simulink model "ejer1"  (R2015b)
settings: Solver=VariableStepAuto  StartTime=0.0  StopTime=10.0  RelTol=1e-3
libraries: powerlib x8
settings Model: Creator=xmax1946  LastModifiedBy=xmax1946

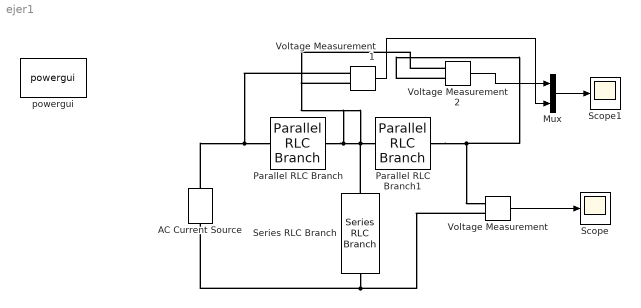
== system ejer1 ==
  AC Current Source : powerlib/Electrical Sources/AC Current Source  Amplitude=1  Phase=0  Frequency=.159  SampleTime=0  Measurements=None
  Mux : Mux  Inputs=2
  Parallel RLC Branch : powerlib/Elements/Parallel RLC Branch  LConnTagsString=a  RConnTagsString=__new0  BranchType=RC  Resistance=10  Inductance=1e-3  SetiL0=off  InitialCurrent=0  Capacitance=1  Setx0=on  InitialVoltage=100  Measurements=None
  Parallel RLC Branch1 : powerlib/Elements/Parallel RLC Branch  LConnTagsString=a  RConnTagsString=__new0  BranchType=RC  Resistance=1  Inductance=1e-3  SetiL0=off  InitialCurrent=0  Capacitance=2  Setx0=on  InitialVoltage=1  Measurements=None
  Scope : Scope
  Scope1 : Scope
  Series RLC Branch : powerlib/Elements/Series RLC Branch  LConnTagsString=__new0  RConnTagsString=__new0  BranchType=R  Resistance=1  Inductance=1e-3  SetiL0=off  InitialCurrent=0  Capacitance=1e-6  Setx0=off  InitialVoltage=0  Measurements=None
  Voltage Measurement : powerlib/Measurements/Voltage Measurement  PhasorSimulation=off  OutputType=Complex  PSBequivalent=0
  Voltage Measurement1 : powerlib/Measurements/Voltage Measurement  PhasorSimulation=off  OutputType=Complex  PSBequivalent=0
  Voltage Measurement2 : powerlib/Measurements/Voltage Measurement  PhasorSimulation=off  OutputType=Complex  PSBequivalent=0
  powergui : powerlib/powergui  Priority=1  SimulationMode=Discrete  SolverType=Tustin/Backward Euler (TBE)  SampleTime=50e-6  frequency=60  SPID=off  DisableSnubberDevices=off  DisableRonSwitches=off  DisableVfSwitches=off  SwTol=0  DisplayEquations=off  Interpol=off  ExternalGateDelay=off  methode=off  Ts=10  FunctionMessages=off  echomessages=off  HookPort=off  EnableUseOfTLC=off  x0status=blocks  frequencyindice=0.159  Pbase=100e6  ErrMax=1e-4  Iterations=50  UnitsV=kV  UnitsW=MW  buscounter=0  RestoreLinks=warning  ResistiveCurrentMeasurement=off  Frange=[0:2:500]  Ylog=off  Xlog=on  ShowGrid=off  save=off  variable=ZData  structure=0  ZoomFFT=off  StartTime=0.0  cycles=1  DisplayStyle=1  fundamental=60  FreqAxis=off  MaxFrequency=1000  frequencyindicesteady=1  RmsSteady=1  display=off
  wires:
  Voltage Measurement/1 -> Scope/1
  Voltage Measurement2/1 -> Mux/1
  Voltage Measurement1/1 -> Mux/2
  Mux/1 -> Scope1/1
  connections:
  AC Current Source/RConn1 -- Voltage Measurement1/LConn1 -- Parallel RLC Branch/LConn1
  Parallel RLC Branch/RConn1 -- Voltage Measurement1/LConn2 -- Voltage Measurement2/LConn1 -- Series RLC Branch/LConn1 -- Parallel RLC Branch1/LConn1
  Series RLC Branch/RConn1 -- AC Current Source/LConn1 -- Voltage Measurement/LConn2
  Parallel RLC Branch1/RConn1 -- Voltage Measurement2/LConn2 -- Voltage Measurement/LConn1
